simulink model "PID_Simulation_System_B"  (R2018b)
settings: Solver=VariableStepAuto  StartTime=0.0  StopTime=60  RelTol=1e-3
undefined symbols (not defined in the file): h, k, k_noise, k_pertub, kd, ki, kp, p1, p2, Pertub, t_pertub
settings Model: Creator=fred  LastModifiedBy=fredericovaz
settings HardwareCC: ProdBitPerLong=64  ProdHWDeviceType=Intel->x86-64 (Linux 64)

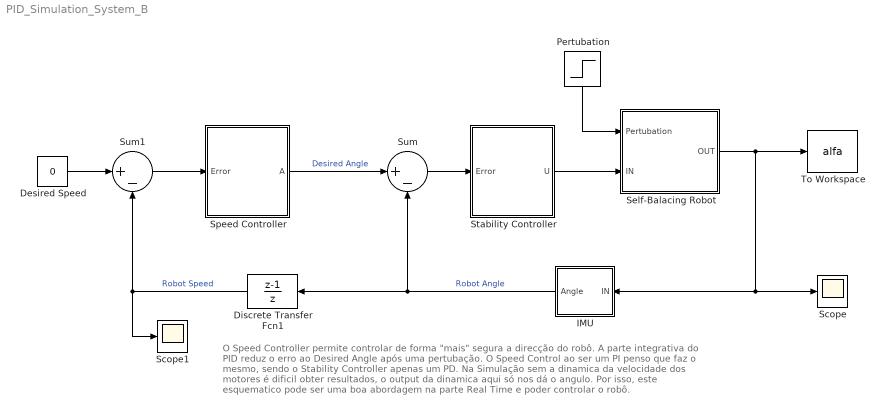
== system PID_Simulation_System_B ==
  note: O Speed Controller permite controlar de forma "mais" segura a direcção do robô.
      | A parte integrativa do PID reduz o erro ao Desired Angle após uma pertubação.
      | O Speed Control ao ser um PI penso que faz o mesmo, sendo o Stability Controller apenas um PD.
      | Na Simulação sem a dinamica da velocidade dos motores é dificil obter resultados, o output da dinamica aqui só nos dá o angulo.
      | Por isso, este esquematico pode ser uma boa abordagem na parte Real Time e poder controlar o robô.
  "Desired Speed " : Constant  Value=0
  Discrete Transfer Fcn1 : DiscreteTransferFcn  Numerator=[1 -1]  Denominator=[1 0]  SampleTime=h
  IMU : Subsystem
  Pertubation : Step  Time=t_pertub  After=Pertub  SampleTime=h
  Scope : Scope
  Scope1 : Scope
  Self-Balacing Robot : Subsystem
  Speed Controller : Subsystem
  Stability Controller : Subsystem
  Sum : Sum  Inputs=|+-
  Sum1 : Sum  Inputs=|+-
  To Workspace : ToWorkspace  VariableName=alfa  SaveFormat=Timeseries  SampleTime=-1
      settings: Save2DSignal=2-D array (concatenate along first dimension)
  wires:
  IMU/1(Angle) -> Discrete Transfer Fcn1/1, Sum/2  "Robot Angle"
  Self-Balacing Robot/1(OUT) -> To Workspace/1, Scope/1, IMU/1(IN)
  Sum/1 -> Stability Controller/1(Error)
  Stability Controller/1(U) -> Self-Balacing Robot/2(IN)
  Pertubation/1 -> Self-Balacing Robot/1(Pertubation)
  Speed Controller/1(A) -> Sum/1  "Desired Angle"
  Sum1/1 -> Speed Controller/1(Error)
  "Desired Speed "/1 -> Sum1/1
  Discrete Transfer Fcn1/1 -> Scope1/1, Sum1/2  "Robot Speed"

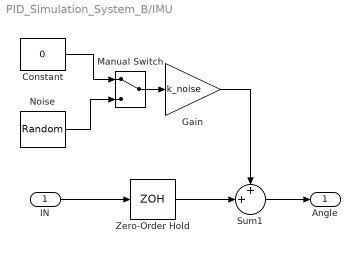
== system PID_Simulation_System_B/IMU ==
  IN : Inport
  Constant : Constant  Value=0
  Gain : Gain  Gain=k_noise
  Manual Switch : ManualSwitch
  Noise : UniformRandomNumber  Minimum=-0.1  Maximum=0.1  SampleTime=h
  Sum1 : Sum  Inputs=++|
  Zero-Order Hold : ZeroOrderHold  SampleTime=h
  Angle : Outport
  wires:
  IN/1 -> Zero-Order Hold/1
  Constant/1 -> Manual Switch/1
  Noise/1 -> Manual Switch/2
  Manual Switch/1 -> Gain/1
  Gain/1 -> Sum1/1
  Zero-Order Hold/1 -> Sum1/2
  Sum1/1 -> Angle/1

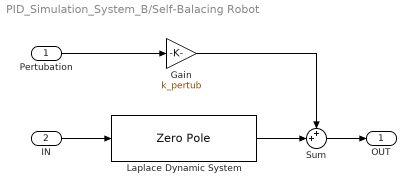
== system PID_Simulation_System_B/Self-Balacing Robot ==
  Pertubation : Inport
  IN : Inport  Port=2
  Gain : Gain  Gain=k_pertub
  Laplace Dynamic System : ZeroPole  Zeros=[ ]  Poles=[ p1 p2 ]  Gain=k
  Sum : Sum  Inputs=++|
  OUT : Outport
  wires:
  Pertubation/1 -> Gain/1
  Laplace Dynamic System/1 -> Sum/2
  Gain/1 -> Sum/1
  IN/1 -> Laplace Dynamic System/1
  Sum/1 -> OUT/1

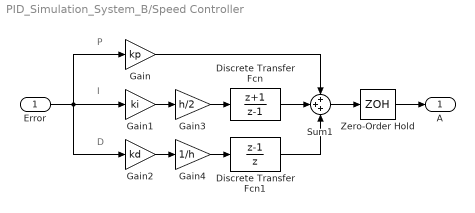
== system PID_Simulation_System_B/Speed Controller ==
  note: I
  note: D
  note: P
  Error : Inport
  Discrete Transfer Fcn : DiscreteTransferFcn  Numerator=[1 +1]  Denominator=[1 -1]  SampleTime=h
  Discrete Transfer Fcn1 : DiscreteTransferFcn  Numerator=[1 -1]  Denominator=[1 0]  SampleTime=h
  Gain : Gain  Gain=kp
  Gain1 : Gain  Gain=ki
  Gain2 : Gain  Gain=kd
  Gain3 : Gain  Gain=h/2
  Gain4 : Gain  Gain=1/h
  Sum1 : Sum  Inputs=+++
  Zero-Order Hold : ZeroOrderHold  SampleTime=h
  A : Outport
  wires:
  Gain1/1 -> Gain3/1
  Error/1 -> Gain1/1, Gain2/1, Gain/1
  Zero-Order Hold/1 -> A/1
  Sum1/1 -> Zero-Order Hold/1
  Gain2/1 -> Gain4/1
  Gain/1 -> Sum1/1
  Gain3/1 -> Discrete Transfer Fcn/1
  Discrete Transfer Fcn/1 -> Sum1/2
  Gain4/1 -> Discrete Transfer Fcn1/1
  Discrete Transfer Fcn1/1 -> Sum1/3

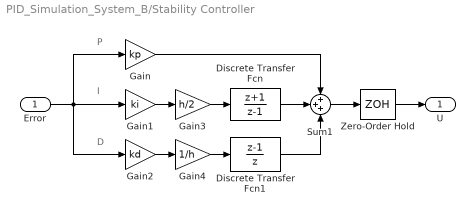
== system PID_Simulation_System_B/Stability Controller ==
  note: I
  note: D
  note: P
  Error : Inport
  Discrete Transfer Fcn : DiscreteTransferFcn  Numerator=[1 +1]  Denominator=[1 -1]  SampleTime=h
  Discrete Transfer Fcn1 : DiscreteTransferFcn  Numerator=[1 -1]  Denominator=[1 0]  SampleTime=h
  Gain : Gain  Gain=kp
  Gain1 : Gain  Gain=ki
  Gain2 : Gain  Gain=kd
  Gain3 : Gain  Gain=h/2
  Gain4 : Gain  Gain=1/h
  Sum1 : Sum  Inputs=+++
  Zero-Order Hold : ZeroOrderHold  SampleTime=h
  U : Outport
  wires:
  Gain1/1 -> Gain3/1
  Error/1 -> Gain1/1, Gain2/1, Gain/1
  Zero-Order Hold/1 -> U/1
  Sum1/1 -> Zero-Order Hold/1
  Gain2/1 -> Gain4/1
  Gain/1 -> Sum1/1
  Gain3/1 -> Discrete Transfer Fcn/1
  Discrete Transfer Fcn/1 -> Sum1/2
  Gain4/1 -> Discrete Transfer Fcn1/1
  Discrete Transfer Fcn1/1 -> Sum1/3
